simulink model "simply13"  (R2021a)
settings: Solver=VariableStepAuto  StartTime=0.0  StopTime=10.0  RelTol=1e-3
libraries: simulink x12, pid_lib x1
settings Model: Creator=O1  LastModifiedBy=O1

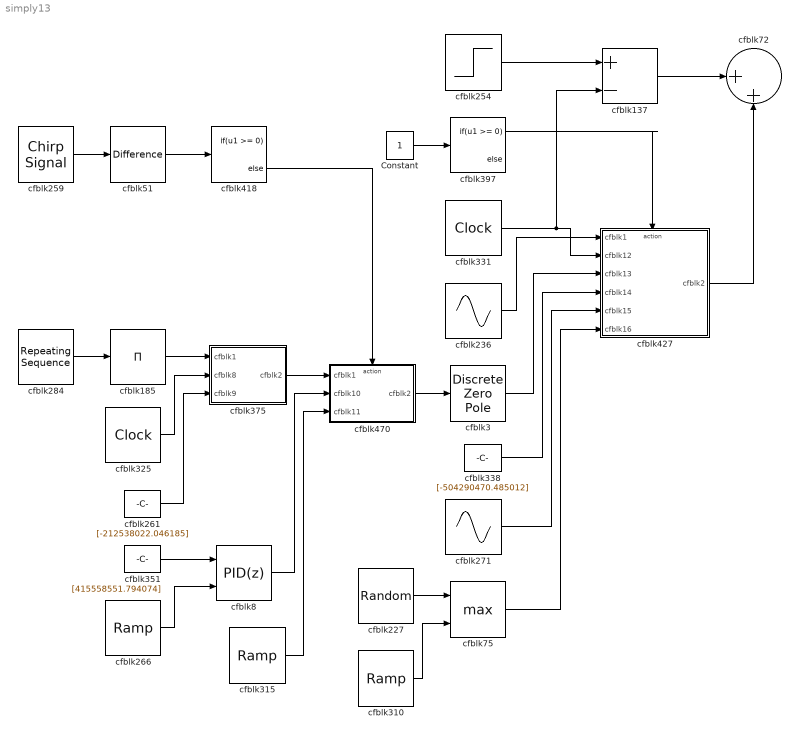
== system simply13 ==
  Constant : Constant
  cfblk137 : Sum  Inputs=+-
  cfblk185 : Product  Inputs=*
  cfblk227 : RandomNumber  Mean=[-34488.154122]  Variance=[75351.385843]  Seed=[84700931.000000]  SampleTime=0.1
  cfblk236 : Sin  Amplitude=[-35405318.481992]  Bias=[-841973075.323358]  SampleTime=0
  cfblk254 : Step  Time=[2.000000]  Before=[801221138.121829]  After=[-89823733.021611]  SampleTime=0
  cfblk259 : simulink/Sources/Chirp Signal  f1=[-775466683.876898]  T=[-642594423.119325]  f2=[-452364156.203623]
  cfblk261 : Constant  Value=[-212538022.046185]  SampleTime=1
  cfblk266 : simulink/Sources/Ramp  slope=[5962.644827]  start=[49.273202]  InitialOutput=[566236.789685]
  cfblk271 : Sin  Amplitude=[-921373321.042865]  Bias=[632755603.310922]  SampleTime=0
  cfblk284 : simulink/Sources/Repeating Sequence  rep_seq_t=[0 2]  rep_seq_y=[229603743.666424, 388280126.205226]
  cfblk3 : DiscreteZeroPole  Poles=[0 0.5]  Gain=1
  cfblk310 : simulink/Sources/Ramp  slope=[3689.412226]  start=[46.253601]  InitialOutput=[-250282.865254]
  cfblk315 : simulink/Sources/Ramp  slope=[-8390.431522]  start=[21.116763]  InitialOutput=[-136585.593152]
  cfblk325 : DigitalClock
  cfblk331 : DigitalClock
  cfblk338 : Constant  Value=[-504290470.485012]  SampleTime=1
  cfblk351 : Constant  Value=[415558551.794074]  SampleTime=1
  cfblk375 : Subsystem
  cfblk397 : If  IfExpression=u1 >= 0  SampleTime=1
  cfblk418 : If  IfExpression=u1 >= 0  SampleTime=1
  cfblk427 : Subsystem  TreatAsAtomicUnit=on
  cfblk470 : Subsystem  TreatAsAtomicUnit=on
  cfblk51 : simulink/Discrete/Difference  ICPrevInput=0.0  OutMin=[]  OutMax=[]  OutDataTypeStr=Inherit: Inherit via back propagation  OutDataType=fixdt(1, 16)  OutScaling=2^-10  DoSatur=off
  cfblk72 : Sum  Inputs=|++
  cfblk75 : MinMax  Function=max  Inputs=2
  cfblk8 : pid_lib/PID Controller (2DOF)  Controller=PID  Form=Parallel  TimeDomain=Discrete-time  UseExternalTs=off  SampleTime=1  IntegratorMethod=Forward Euler  FilterMethod=Forward Euler  ControllerParametersSource=internal  P=1  I=1  D=0  UseFilter=on  N=100  b=1  c=1  TunerSelectOption=Transfer Function Based (PID Tuner App)  InitialConditionSource=internal  InitialConditionForIntegrator=0  InitialConditionForFilter=0  DifferentiatorICPrevScaledInput=0  ExternalReset=none  TrackingMode=off  Kt=1  LimitOutput=off  SatLimitsSource=internal  UpperSaturationLimit=inf  LowerSaturationLimit=-inf  LinearizeAsGain=off  AntiWindupMode=none  Kb=1  POutMin=[]  POutMax=[]  IOutMin=[]  IOutMax=[]  DOutMin=[]  DOutMax=[]  NOutMin=[]  NOutMax=[]  bOutMin=[]  bOutMax=[]  cOutMin=[]  cOutMax=[]  SumOutMin=[]  SumOutMax=[]  SaturationOutMin=[]  SaturationOutMax=[]  PParamMin=[]  PParamMax=[]  IParamMin=[]  IParamMax=[]  DParamMin=[]  DParamMax=[]  NParamMin=[]  NParamMax=[]  bParamMin=[]  bParamMax=[]  cParamMin=[]  cParamMax=[]  KbParamMin=[]  KbParamMax=[]  KtParamMin=[]  KtParamMax=[]  KbOutMin=[]  KbOutMax=[]  KtOutMin=[]  KtOutMax=[]  IntegratorOutMin=[]  IntegratorOutMax=[]  FilterOutMin=[]  FilterOutMax=[]  SumI1OutMin=[]  SumI1OutMax=[]  SumI2OutMin=[]  SumI2OutMax=[]  SumI3OutMin=[]  SumI3OutMax=[]  SumI4OutMin=[]  SumI4OutMax=[]  SumDOutMin=[]  SumDOutMax=[]  Sum1OutMin=[]  Sum1OutMax=[]  Sum2OutMin=[]  Sum2OutMax=[]  Sum3OutMin=[]  Sum3OutMax=[]  DifferentiatorOutMin=[]  DifferentiatorOutMax=[]  FilterDiffOutCoefMin=[]  FilterDiffOutCoefMax=[]  ReciprocalOutMin=[]  ReciprocalOutMax=[]  SumDenOutMin=[]  SumDenOutMax=[]  SumNumOutMin=[]  SumNumOutMax=[]  DivideOutMin=[]  DivideOutMax=[]  UdiffTsProdOutMin=[]  UdiffTsProdOutMax=[]  NTsProdOutMin=[]  NTsProdOutMax=[]  UintegralTsProdOutMin=[]  UintegralTsProdOutMax=[]  UngainTsProdOutMin=[]  UngainTsProdOutMax=[]  IntegratorContinuousStateAttributes=''  IntegratorStateMustResolveToSignalObject=off  IntegratorRTWStateStorageClass=Auto  FilterContinuousStateAttributes=''  FilterStateMustResolveToSignalObject=off  FilterRTWStateStorageClass=Auto  ParallelPVariant=InternalParameters  IdealPVariant=Disabled  IVariant=InternalParameters  DVariant=InternalParameters  bVariant=InternalParameters  cVariant=InternalParameters  IntegratorVariant=Discrete  SatVariant=Disabled  AWVariant=Passthrough  PCopyVariant=Disabled  TRVariant=Disabled  FdbkBlocksVariant=Forward  IdealPFdbkVariant=Disabled  SatFdbkVariant=Disabled  DerivativeFilterVariant=ForwardEulerFilter  NVariant=InternalParameters  NCopyVariant=Disabled  FilterICVariant=InternalICsFilter  IntegratorICVariant=InternalICs  ExternalResetVariant=Disabled  TRSumVariant=Passthrough  SumFdbkVariant=Disabled  SumVariant=Sum_PID  TsampFilterVariant=InternalTs  TsampNgainVariant=Passthrough  TsampIntegralVariant=Passthrough  ExternalSaturationOutDataTypeStr=Inherit: Same as second input
      settings: SourceProductBaseCode=SL
  wires:
  cfblk266/1 -> cfblk8/2
  cfblk470/1(cfblk2) -> cfblk3/1
  cfblk259/1 -> cfblk51/1
  cfblk185/1 -> cfblk375/1(cfblk1)
  cfblk51/1 -> cfblk418/1
  cfblk351/1 -> cfblk8/1
  cfblk418/2 -> cfblk470/Action
  cfblk284/1 -> cfblk185/1
  cfblk375/1(cfblk2) -> cfblk470/1(cfblk1)
  cfblk261/1 -> cfblk375/3(cfblk9)
  cfblk325/1 -> cfblk375/2(cfblk8)
  cfblk8/1 -> cfblk470/2(cfblk10)
  cfblk315/1 -> cfblk470/3(cfblk11)
  cfblk3/1 -> cfblk427/3(cfblk13)
  cfblk338/1 -> cfblk427/4(cfblk14)
  cfblk271/1 -> cfblk427/5(cfblk15)
  cfblk427/1(cfblk2) -> cfblk72/2
  cfblk75/1 -> cfblk427/6(cfblk16)
  cfblk227/1 -> cfblk75/1
  Constant/1 -> cfblk397/1
  cfblk236/1 -> cfblk427/1(cfblk1)
  cfblk397/1 -> cfblk427/Action
  cfblk254/1 -> cfblk137/1
  cfblk137/1 -> cfblk72/1
  cfblk310/1 -> cfblk75/2
  cfblk331/1 -> cfblk137/2, cfblk427/2(cfblk12)

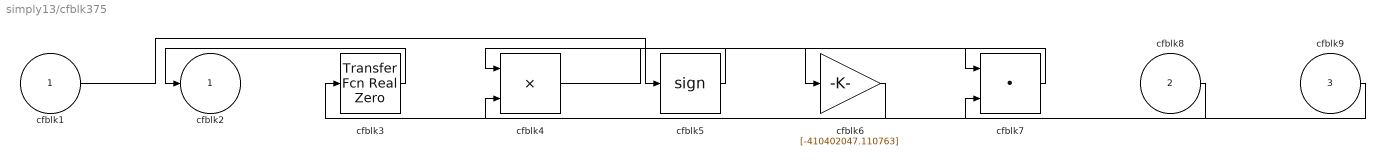
== system simply13/cfblk375 ==
  cfblk1 : Inport
  cfblk8 : Inport  Port=2
  cfblk9 : Inport  Port=3
  cfblk3 : simulink/Discrete/Transfer Fcn Real Zero  ZeroZ=0.75  ICPrevInput=0.0  DoSatur=off
      settings: SourceProductBaseCode=SL
  cfblk4 : Product
  cfblk5 : Signum
  cfblk6 : Gain  Gain=[-410402047.110763]
  cfblk7 : DotProduct  InputSameDT=on  OutDataTypeStr=Inherit: Inherit via internal rule
  cfblk2 : Outport
  wires:
  cfblk7/1 -> cfblk6/1
  cfblk3/1 -> cfblk2/1
  cfblk6/1 -> cfblk3/1
  cfblk1/1 -> cfblk5/1
  cfblk4/1 -> cfblk7/1
  cfblk8/1 -> cfblk7/2
  cfblk5/1 -> cfblk4/1
  cfblk9/1 -> cfblk4/2

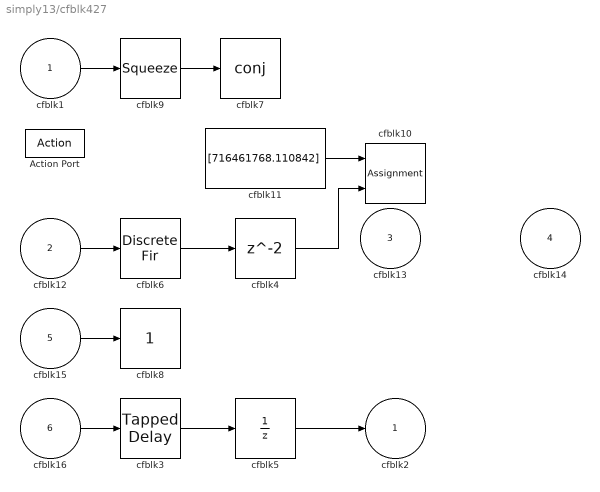
== system simply13/cfblk427 ==
  cfblk1 : Inport
  cfblk12 : Inport  Port=2
  cfblk13 : Inport  Port=3
  cfblk14 : Inport  Port=4
  cfblk15 : Inport  Port=5
  cfblk16 : Inport  Port=6
  Action Port : ActionPort  ActionPortLabel=if(u1 >= 0)
  cfblk10 : Assignment  DiagnosticForDimensions=Warning  IndexOptions=Index vector (dialog)  Indices=1  OutputSizes=1
  cfblk11 : Constant  Value=[716461768.110842]  SampleTime=1
  cfblk3 : simulink/Discrete/Tapped Delay  vinit=0.0  samptime=-1  NumDelays=1  DelayOrder=Oldest  includeCurrent=off
  cfblk4 : Delay
  cfblk5 : UnitDelay  SampleTime=-1  HasFrameUpgradeWarning=on
  cfblk6 : DiscreteFir
  cfblk7 : Math  Operator=conj  SaturateOnIntegerOverflow=on
  cfblk8 : simulink/Math Operations/Slider Gain  gain=1  low=0  high=2
  cfblk9 : Squeeze
  cfblk2 : Outport
  wires:
  cfblk15/1 -> cfblk8/1
  cfblk4/1 -> cfblk10/2
  cfblk11/1 -> cfblk10/1
  cfblk3/1 -> cfblk5/1
  cfblk5/1 -> cfblk2/1
  cfblk12/1 -> cfblk6/1
  cfblk16/1 -> cfblk3/1
  cfblk1/1 -> cfblk9/1
  cfblk6/1 -> cfblk4/1
  cfblk9/1 -> cfblk7/1

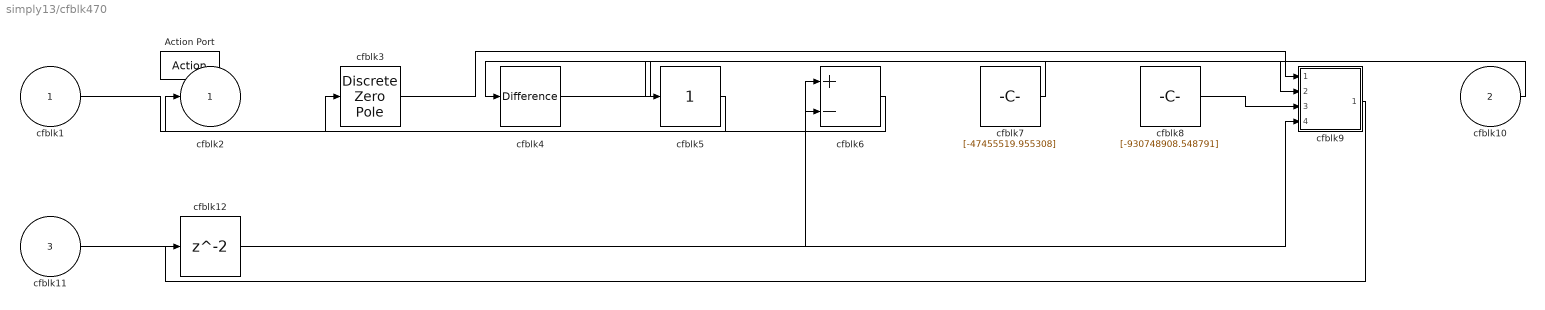
== system simply13/cfblk470 ==
  cfblk1 : Inport
  cfblk10 : Inport  Port=2
  cfblk11 : Inport  Port=3
  Action Port : ActionPort  ActionPortLabel=else
  cfblk12 : Delay
  cfblk3 : DiscreteZeroPole  Poles=[0 0.5]  Gain=1  SampleTime=-1
  cfblk4 : simulink/Discrete/Difference  ICPrevInput=0.0  OutMin=[]  OutMax=[]  OutDataTypeStr=Inherit: Inherit via back propagation  OutDataType=fixdt(1, 16)  OutScaling=2^-10  DoSatur=off
  cfblk5 : simulink/Math Operations/Slider Gain  gain=1  low=0  high=2
  cfblk6 : Sum  Inputs=+-
  cfblk7 : Constant  Value=[-47455519.955308]  SampleTime=1
  cfblk8 : Constant  Value=[-930748908.548791]  SampleTime=1
  cfblk9 : Subsystem
  cfblk2 : Outport
  wires:
  cfblk7/1 -> cfblk4/1
  cfblk6/1 -> cfblk3/1
  cfblk5/1 -> cfblk2/1
  cfblk3/1 -> cfblk9/1(cfblk1)
  cfblk4/1 -> cfblk9/2(cfblk13)
  cfblk8/1 -> cfblk9/3(cfblk14)
  cfblk1/1 -> cfblk6/1
  cfblk10/1 -> cfblk5/1
  cfblk11/1 -> cfblk9/4(cfblk15)
  cfblk9/1(cfblk2) -> cfblk12/1
  cfblk12/1 -> cfblk6/2

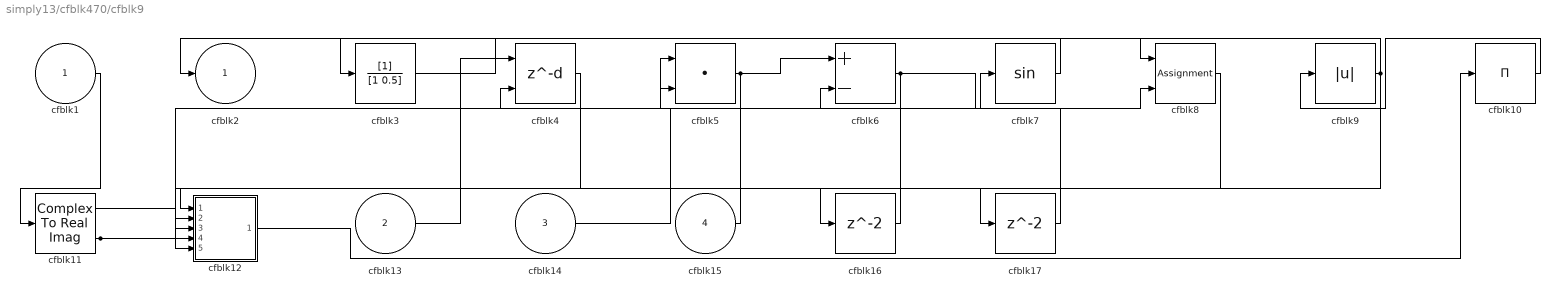
== system simply13/cfblk470/cfblk9 ==
  cfblk1 : Inport
  cfblk13 : Inport  Port=2
  cfblk14 : Inport  Port=3
  cfblk15 : Inport  Port=4
  cfblk10 : Product  Inputs=*
  cfblk11 : ComplexToRealImag
  cfblk12 : Subsystem
  cfblk16 : Delay
  cfblk17 : Delay
  cfblk3 : DiscreteFilter
  cfblk4 : Delay  DelayLengthSource=Input port
      settings: InputPortMap=u0,p1
  cfblk5 : DotProduct  InputSameDT=on  OutDataTypeStr=Inherit: Inherit via internal rule
  cfblk6 : Sum  Inputs=+-
  cfblk7 : Trigonometry
  cfblk8 : Assignment  DiagnosticForDimensions=Warning  IndexOptions=Index vector (dialog)  Indices=1  OutputSizes=1
  cfblk9 : Abs
  cfblk2 : Outport
  wires:
  cfblk13/1 -> cfblk4/1
  cfblk12/1(cfblk2) -> cfblk10/1
  cfblk15/1 -> cfblk5/1
  cfblk9/1 -> cfblk2/1, cfblk16/1
  cfblk11/1 -> cfblk4/2
  cfblk3/1 -> cfblk8/1
  cfblk14/1 -> cfblk7/1
  cfblk11/2 -> cfblk5/2, cfblk12/4(cfblk15)
  cfblk10/1 -> cfblk9/1
  cfblk7/1 -> cfblk3/1
  cfblk1/1 -> cfblk11/1
  cfblk6/1 -> cfblk8/2, cfblk12/5(cfblk16)
  cfblk5/1 -> cfblk6/1, cfblk12/3(cfblk14)
  cfblk4/1 -> cfblk12/2(cfblk13)
  cfblk16/1 -> cfblk12/1(cfblk1)
  cfblk8/1 -> cfblk17/1
  cfblk17/1 -> cfblk6/2

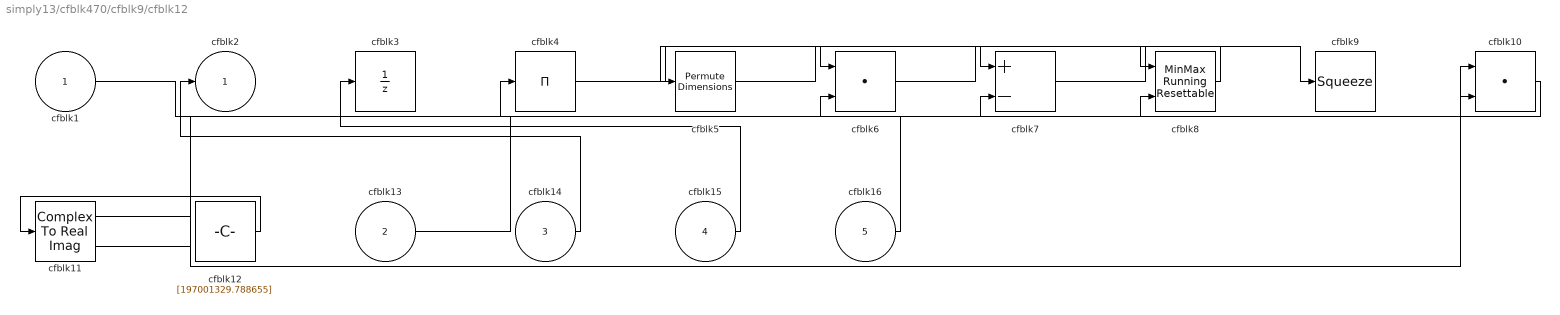
== system simply13/cfblk470/cfblk9/cfblk12 ==
  cfblk1 : Inport
  cfblk13 : Inport  Port=2
  cfblk14 : Inport  Port=3
  cfblk15 : Inport  Port=4
  cfblk16 : Inport  Port=5
  cfblk10 : DotProduct  InputSameDT=on  OutDataTypeStr=Inherit: Inherit via internal rule
  cfblk11 : ComplexToRealImag
  cfblk12 : Constant  Value=[197001329.788655]  SampleTime=1
  cfblk3 : UnitDelay  SampleTime=-1  HasFrameUpgradeWarning=on
  cfblk4 : Product  Inputs=*
  cfblk5 : PermuteDimensions
  cfblk6 : DotProduct  InputSameDT=on  OutDataTypeStr=Inherit: Inherit via internal rule
  cfblk7 : Sum  Inputs=+-
  cfblk8 : simulink/Math Operations/MinMax Running Resettable  Function=min  vinit=0.0
  cfblk9 : Squeeze
  cfblk2 : Outport
  wires:
  cfblk16/1 -> cfblk4/1
  cfblk15/1 -> cfblk3/1
  cfblk7/1 -> cfblk9/1
  cfblk4/1 -> cfblk6/1
  cfblk14/1 -> cfblk2/1
  cfblk12/1 -> cfblk11/1
  cfblk13/1 -> cfblk6/2
  cfblk11/1 -> cfblk10/1
  cfblk5/1 -> cfblk7/1
  cfblk6/1 -> cfblk8/1
  cfblk1/1 -> cfblk7/2
  cfblk8/1 -> cfblk5/1
  cfblk11/2 -> cfblk10/2
  cfblk10/1 -> cfblk8/2
